simulink library "TrueDurationTime"  (R2019b)
settings: Solver=VariableStepAuto  StartTime=0.0  StopTime=10.0  RelTol=1e-3
settings Model: Creator=GW00167954  LastModifiedBy=GW00167954

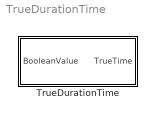
== system TrueDurationTime ==
  TrueDurationTime : Subsystem  mask(TrueDurationTime){TCycle=0.02}
      mask prompts: TCycle "CycleTime"
      mask help:
      | Calculate the truth duration time.You should set the physical value of the model's cycle time.
      | BooleanValue : DataType:Boolean Dimension:1

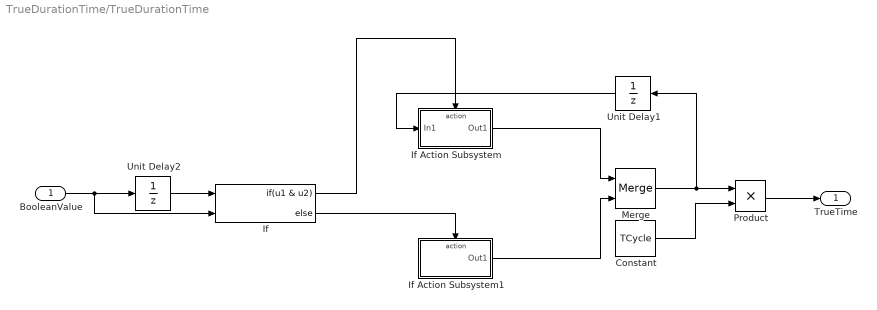
== system TrueDurationTime/TrueDurationTime ==
  BooleanValue : Inport  OutDataTypeStr=boolean
  Constant : Constant  Value=TCycle  OutDataTypeStr=single
  If : If  NumInputs=2  IfExpression=u1 & u2
  If Action Subsystem : Subsystem  TreatAsAtomicUnit=on
  If Action Subsystem1 : Subsystem  TreatAsAtomicUnit=on
  Merge : Merge
  Product : Product
  Unit Delay1 : UnitDelay  SampleTime=-1  HasFrameUpgradeWarning=on
  Unit Delay2 : UnitDelay  SampleTime=-1  HasFrameUpgradeWarning=on
  TrueTime : Outport  OutDataTypeStr=single
  wires:
  If Action Subsystem1/1(Out1) -> Merge/2
  If Action Subsystem/1(Out1) -> Merge/1
  Constant/1 -> Product/2
  BooleanValue/1 -> If/2, Unit Delay2/1
  Merge/1 -> Unit Delay1/1, Product/1
  If/1 -> If Action Subsystem/Action
  If/2 -> If Action Subsystem1/Action
  Unit Delay1/1 -> If Action Subsystem/1(In1)
  Product/1 -> TrueTime/1
  Unit Delay2/1 -> If/1

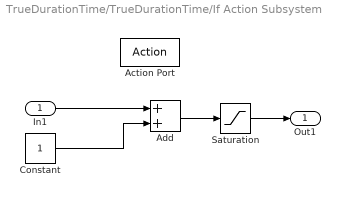
== system TrueDurationTime/TrueDurationTime/If Action Subsystem ==
  In1 : Inport
  Action Port : ActionPort
  Add : Sum  OutDataTypeStr=uint16
  Constant : Constant  OutDataTypeStr=uint16
  Saturation : Saturate  UpperLimit=60000  LowerLimit=0
  Out1 : Outport
  wires:
  In1/1 -> Add/1
  Add/1 -> Saturation/1
  Constant/1 -> Add/2
  Saturation/1 -> Out1/1

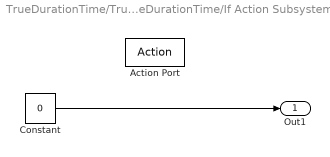
== system TrueDurationTime/TrueDurationTime/If Action Subsystem1 ==
  Action Port : ActionPort
  Constant : Constant  Value=0  OutDataTypeStr=uint16
  Out1 : Outport
  wires:
  Constant/1 -> Out1/1
